simulink model "flightControlSystem - Copy"  (R2024b)
settings: Solver=ode3  StartTime=0  StopTime=TFinal  FixedStep=Ts  RelTol=1e-3  EnableMultiTasking=on
undefined symbols (not defined in the file): codertarget, Controller, DiscIntNeverNeededParam, Discrete, Estimator, g, gray, init, orient_ref, pos_ref, Sensors, Time, Ts, var_acc_angle_N, var_bias_gyr_N, var_gyro_p_N, Vehicle
libraries: simulink x54, matrix_library x7, slpidlib x4, ctrlSharedLib x4, sharedtransform x3, parrotlib x2
(part 3 of 3)

== matlab function flightControlSystem - Copy/Image Processing System/MATLAB Function ==
  data: R input; BW output; G input; B input
function BW =createGreenLineMask(R,G,B)
%createMask  Threshold RGB image using auto-generated code from colorThresholder app.
%  [BW,MASKEDRGBIMAGE] = createMask(RGB) thresholds image RGB using
%  auto-generated code from the colorThresholder app. The colorspace and
%  range for each channel of the colorspace were set within the app. The
%  segmentation mask is returned in BW, and a composite of the mask and
%  original RGB images is returned in maskedRGBImage.

% Auto-generated by colorThresholder app on 05-Feb-2024 
%------------------------------------------------------


% Define thresholds for channel 1 based on histogram settings
%channel1Min = 185.000;
%channel1Max = 221.000;

% Define thresholds for channel 2 based on histogram settings
%channel2Min = 209.000;
%channel2Max = 247.000;

% Define thresholds for channel 3 based on histogram settings

%channel3Min = 132.000;
%channel3Max=195.000;

% Define thresholds for channel 1 based on histogram settings
%channel1Min = 148.000;
%channel1Max = 207.000;

% Define thresholds for channel 2 based on histogram settings
%channel2Min = 188.000;
%channel2Max = 223.000;

% Define thresholds for channel 3 based on histogram settings
%channel3Min = 127.000;
%channel3Max = 180.000;
% Define thresholds for channel 1 based on histogram settings
channel1Min = 149.000;
channel1Max = 206.000;

% Define thresholds for channel 2 based on histogram settings
channel2Min = 186.000;
channel2Max = 228.000;

% Define thresholds for channel 3 based on histogram settings
channel3Min = 118.000;
channel3Max = 177.000;


% Create mask based on chosen histogram thresholds
sliderBW = (R >= channel1Min ) & (R <= channel1Max) & ...
    (G >= channel2Min ) & (G <= channel2Max) & ...
    (B >= channel3Min ) & (B <= channel3Max);
BW = sliderBW;


end

== matlab function flightControlSystem - Copy/Flight Control System/Controller/Position Controller/Position error transformation (Earth to Body frame) ==
  data: yaw input; xy_err_earth input; xy_err_body output
function xy_err_body = fcn(yaw,xy_err_earth)

transformation = [cos(yaw), sin(yaw); -sin(yaw),  cos(yaw)];
xy_err_body = transformation * xy_err_earth;


end

== stateflow chart flightControlSystem - Copy/Flight Control System/Path Planning/Chart ==
  state FindingLineLeft
    during:
    yawOut=yawOut-0.001;
  state TakeOff
    during:
    xout=0;
    yout=0;
    zout=-0.9;
    yawOut=0;
  state YawRight
    during:
    yawOut=yawOut+0.001;
    xout=xout+0.00035*cos(estim_YAW);
    yout=yout+0.00035*sin(estim_YAW);
  state MoveForward
    during:
    xout=xout+0.0005*cos(estim_YAW);
    yout=yout+0.0005*sin(estim_YAW);
  state YawLeft
    during:
    yawOut=yawOut-0.001;
    xout=xout+0.00035*cos(estim_YAW);
    yout=yout+0.00035*sin(estim_YAW);
  state FindingLineRight
    during:
    yawOut=yawOut+0.001
  state Land
    entry:
    zout=-0.1;
    landEnable = true;
  FindingLineLeft -> MoveForward : [up==1]
  TakeOff -> FindingLineLeft [order 1] : [after(3,sec)&&up==0&&LineLeft==1]
  (default) -> TakeOff
  YawRight -> MoveForward : [after(0.5,sec)&&up==1]
  TakeOff -> MoveForward [order 2] : [after(3,sec)&&up==1]
  MoveForward -> YawRight [order 1] : [right==1]
  TakeOff -> Land [order 4] : [after(60,sec)]
  TakeOff -> FindingLineRight [order 3] : [after(3,sec)&&up==0]
  YawLeft -> MoveForward : [after(0.5,sec)&&up==1]
  MoveForward -> YawLeft [order 2] : [left==1]
  FindingLineRight -> MoveForward : [up==1]
  MoveForward -> Land [order 3] : [circle==1&&right==0&&left==0]
  data: yawOut output single; xout output single; estim_YAW input; right input; up input; circle input; left input; LineLeft input; yout output single; zout output single; landEnable output

== stateflow chart flightControlSystem - Copy/Flight Control System/Path Planning/Chart1 ==
  state TakeOff
    during:
    xout=0;
    yout=0;
    zout=-1.1;
  state MoveForward
    during:
    xout=xout+0.0005;
  state Land
    entry:
    landStatusFlag=true;
  (default) -> TakeOff
  TakeOff -> MoveForward : [after(3,sec)&&forward==1]
  MoveForward -> Land : [circle==0&&forward==0]
  data: forward input; circle input; xout output; yout output; zout output; landStatusFlag output boolean =false; yawOut input
